simulink model "W3P1"  (R2020b)
settings: Solver=VariableStepAuto  StartTime=0.0  StopTime=10.0  RelTol=1e-3
settings Model: Creator=ASUS  LastModifiedBy=ASUS

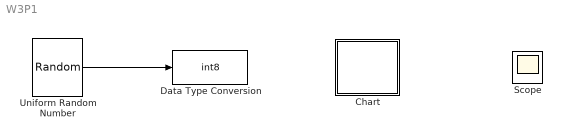
== system W3P1 ==
  Chart : Stateflow chart  TreatAsAtomicUnit=on
  Data Type Conversion : DataTypeConversion  OutDataTypeStr=int8  RndMeth=Nearest
  Scope : Scope
  Uniform Random Number : UniformRandomNumber  SampleTime=0.1
  wires:
  Uniform Random Number/1 -> Data Type Conversion/1

== stateflow chart W3P1/Chart ==
